simulink model "E5_1_Harmonicas"  (R2018a)
settings: Solver=VariableStepAuto  StartTime=0.0  StopTime=1  RelTol=1e-3
libraries: powerlib x109
settings Model: Creator=Rafael Pavan  LastModifiedBy=Rafael Pavan

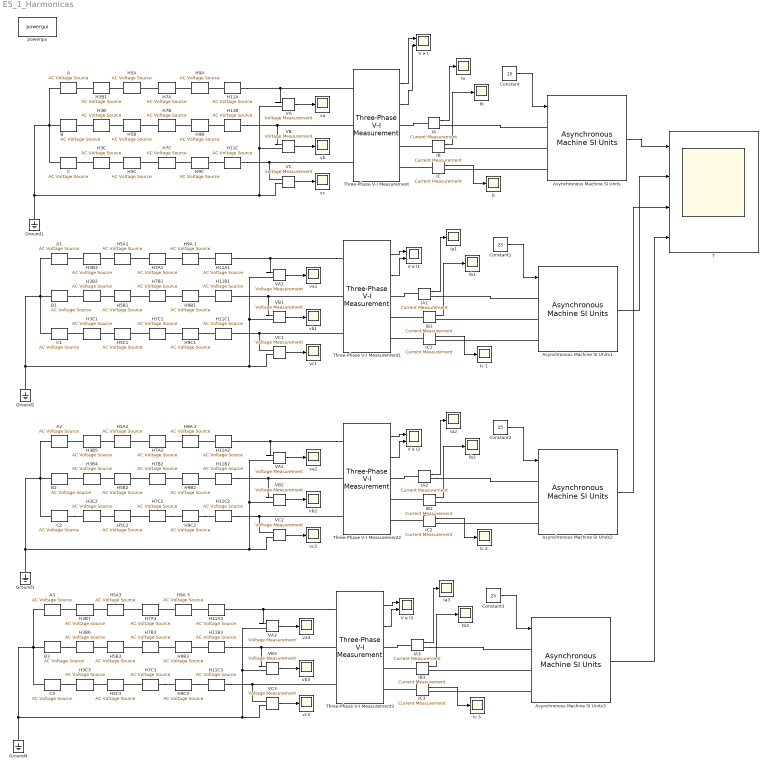
== system E5_1_Harmonicas ==
  A{,1..3} (4 alike) : powerlib/Electrical Sources/AC Voltage Source  Amplitude=179.605  Phase=0  Frequency=60  SampleTime=0  Measurements=None  BusType=PV  Pref=100e4  Qref=0  Qmin=-inf  Qmax=+inf
  Asynchronous Machine SI Units{,1..3} (4 alike) : powerlib/Machines/Asynchronous Machine SI Units  RotorType=Squirrel-cage  PresetModel=No  MechanicalLoad=Torque Tm  ShowDetailedParameters=on  ReferenceFrame=Rotor  Units=SI  MeasurementBus=off  NominalParameters=[38105 220 60]  Stator=[0.5968 0.0003495]  Rotor=[0.6258 0.005473]  Cage1=[0.4155 0.002066]  Cage2=[0.4168 0.0003495]  Lm=0.0354  Mechanical=[0.05 0.005879 3]  PolePairs=2  InitialConditions=[0.03 0 0 0 0 0 0 0]  SimulateSaturation=off  Saturation=[14.03593122, 27.81365428, 53.79336849, 72.68890987, 97.98006896, 148.6815601, 215.7428561, 302.9841135, 428.7778367 ; 230, 322, 414, 460, 506, 552, 598, 644, 690]  LoadFlowParameters=1492000  TsPowergui=0  TsBlock=-1  IterativeModel=Trapezoidal non iterative  IterativeDiscreteModel=Trapezoidal non iterative  Pmec=29150
  B{,1..3} (4 alike) : powerlib/Electrical Sources/AC Voltage Source  Amplitude=179.605  Phase=-120  Frequency=60  SampleTime=0  Measurements=None  BusType=PV  Pref=100e4  Qref=0  Qmin=-inf  Qmax=+inf
  C{,1..3} (4 alike) : powerlib/Electrical Sources/AC Voltage Source  Amplitude=179.605  Phase=120  Frequency=60  SampleTime=0  Measurements=None  BusType=PV  Pref=100e4  Qref=0  Qmin=-inf  Qmax=+inf
  Constant{,1..3} (4 alike) : Constant  Value=25
  Ground{1..4} (4 alike) : powerlib/Elements/Ground  LConnTagsString=a
  H11A : powerlib/Electrical Sources/AC Voltage Source  Amplitude=0  Phase=0  Frequency=660  SampleTime=0  Measurements=None  BusType=PV  Pref=100e4  Qref=0  Qmin=-inf  Qmax=+inf
  H11A1 : powerlib/Electrical Sources/AC Voltage Source  Amplitude=0  Phase=0  Frequency=660  SampleTime=0  Measurements=None  BusType=PV  Pref=100e4  Qref=0  Qmin=-inf  Qmax=+inf
  H11A2 : powerlib/Electrical Sources/AC Voltage Source  Amplitude=179.605*10/100  Phase=0  Frequency=660  SampleTime=0  Measurements=None  BusType=PV  Pref=100e4  Qref=0  Qmin=-inf  Qmax=+inf
  H11A3 : powerlib/Electrical Sources/AC Voltage Source  Amplitude=179.605*5/100  Phase=0  Frequency=660  SampleTime=0  Measurements=None  BusType=PV  Pref=100e4  Qref=0  Qmin=-inf  Qmax=+inf
  H11B : powerlib/Electrical Sources/AC Voltage Source  Amplitude=0  Phase=-120*11  Frequency=660  SampleTime=0  Measurements=None  BusType=PV  Pref=100e4  Qref=0  Qmin=-inf  Qmax=+inf
  H11B1 : powerlib/Electrical Sources/AC Voltage Source  Amplitude=0  Phase=-120*11  Frequency=660  SampleTime=0  Measurements=None  BusType=PV  Pref=100e4  Qref=0  Qmin=-inf  Qmax=+inf
  H11B2 : powerlib/Electrical Sources/AC Voltage Source  Amplitude=179.605*10/100  Phase=-120*11  Frequency=660  SampleTime=0  Measurements=None  BusType=PV  Pref=100e4  Qref=0  Qmin=-inf  Qmax=+inf
  H11B3 : powerlib/Electrical Sources/AC Voltage Source  Amplitude=179.605*5/100  Phase=-120*11  Frequency=660  SampleTime=0  Measurements=None  BusType=PV  Pref=100e4  Qref=0  Qmin=-inf  Qmax=+inf
  H11C : powerlib/Electrical Sources/AC Voltage Source  Amplitude=0  Phase=120*11  Frequency=660  SampleTime=0  Measurements=None  BusType=PV  Pref=100e4  Qref=0  Qmin=-inf  Qmax=+inf
  H11C1 : powerlib/Electrical Sources/AC Voltage Source  Amplitude=0  Phase=120*11  Frequency=660  SampleTime=0  Measurements=None  BusType=PV  Pref=100e4  Qref=0  Qmin=-inf  Qmax=+inf
  H11C2 : powerlib/Electrical Sources/AC Voltage Source  Amplitude=179.605*10/100  Phase=120*11  Frequency=660  SampleTime=0  Measurements=None  BusType=PV  Pref=100e4  Qref=0  Qmin=-inf  Qmax=+inf
  H11C3 : powerlib/Electrical Sources/AC Voltage Source  Amplitude=179.605*5/100  Phase=120*11  Frequency=660  SampleTime=0  Measurements=None  BusType=PV  Pref=100e4  Qref=0  Qmin=-inf  Qmax=+inf
  H3B : powerlib/Electrical Sources/AC Voltage Source  Amplitude=179.605*10/100  Phase=-120*3  Frequency=180  SampleTime=0  Measurements=None  BusType=PV  Pref=100e4  Qref=0  Qmin=-inf  Qmax=+inf
  H3B1 : powerlib/Electrical Sources/AC Voltage Source  Amplitude=179.605*10/100  Phase=0*3  Frequency=60*3  SampleTime=0  Measurements=None  BusType=PV  Pref=100e4  Qref=0  Qmin=-inf  Qmax=+inf
  H3B2 : powerlib/Electrical Sources/AC Voltage Source  Amplitude=0  Phase=-120*3  Frequency=180  SampleTime=0  Measurements=None  BusType=PV  Pref=100e4  Qref=0  Qmin=-inf  Qmax=+inf
  H3B3 : powerlib/Electrical Sources/AC Voltage Source  Amplitude=0  Phase=0*3  Frequency=60*3  SampleTime=0  Measurements=None  BusType=PV  Pref=100e4  Qref=0  Qmin=-inf  Qmax=+inf
  H3B4 : powerlib/Electrical Sources/AC Voltage Source  Amplitude=0  Phase=-120*3  Frequency=180  SampleTime=0  Measurements=None  BusType=PV  Pref=100e4  Qref=0  Qmin=-inf  Qmax=+inf
  H3B5 : powerlib/Electrical Sources/AC Voltage Source  Amplitude=0  Phase=0*3  Frequency=60*3  SampleTime=0  Measurements=None  BusType=PV  Pref=100e4  Qref=0  Qmin=-inf  Qmax=+inf
  H3B6 : powerlib/Electrical Sources/AC Voltage Source  Amplitude=0  Phase=-120*3  Frequency=180  SampleTime=0  Measurements=None  BusType=PV  Pref=100e4  Qref=0  Qmin=-inf  Qmax=+inf
  H3B7 : powerlib/Electrical Sources/AC Voltage Source  Amplitude=0  Phase=0*3  Frequency=60*3  SampleTime=0  Measurements=None  BusType=PV  Pref=100e4  Qref=0  Qmin=-inf  Qmax=+inf
  H3C : powerlib/Electrical Sources/AC Voltage Source  Amplitude=179.605*10/100  Phase=120*3  Frequency=180  SampleTime=0  Measurements=None  BusType=PV  Pref=100e4  Qref=0  Qmin=-inf  Qmax=+inf
  H3C1 : powerlib/Electrical Sources/AC Voltage Source  Amplitude=0  Phase=120*3  Frequency=180  SampleTime=0  Measurements=None  BusType=PV  Pref=100e4  Qref=0  Qmin=-inf  Qmax=+inf
  H3C2 : powerlib/Electrical Sources/AC Voltage Source  Amplitude=0  Phase=120*3  Frequency=180  SampleTime=0  Measurements=None  BusType=PV  Pref=100e4  Qref=0  Qmin=-inf  Qmax=+inf
  H3C3 : powerlib/Electrical Sources/AC Voltage Source  Amplitude=0  Phase=120*3  Frequency=180  SampleTime=0  Measurements=None  BusType=PV  Pref=100e4  Qref=0  Qmin=-inf  Qmax=+inf
  H5A : powerlib/Electrical Sources/AC Voltage Source  Amplitude=0  Phase=0  Frequency=300  SampleTime=0  Measurements=None  BusType=PV  Pref=100e4  Qref=0  Qmin=-inf  Qmax=+inf
  H5A1 : powerlib/Electrical Sources/AC Voltage Source  Amplitude=0  Phase=0  Frequency=300  SampleTime=0  Measurements=None  BusType=PV  Pref=100e4  Qref=0  Qmin=-inf  Qmax=+inf
  H5A2 : powerlib/Electrical Sources/AC Voltage Source  Amplitude=179.605*10/100  Phase=0  Frequency=300  SampleTime=0  Measurements=None  BusType=PV  Pref=100e4  Qref=0  Qmin=-inf  Qmax=+inf
  H5A3 : powerlib/Electrical Sources/AC Voltage Source  Amplitude=179.605*5/100  Phase=0  Frequency=300  SampleTime=0  Measurements=None  BusType=PV  Pref=100e4  Qref=0  Qmin=-inf  Qmax=+inf
  H5B : powerlib/Electrical Sources/AC Voltage Source  Amplitude=0  Phase=-120*5  Frequency=300  SampleTime=0  Measurements=None  BusType=PV  Pref=100e4  Qref=0  Qmin=-inf  Qmax=+inf
  H5B1 : powerlib/Electrical Sources/AC Voltage Source  Amplitude=0  Phase=-120*5  Frequency=300  SampleTime=0  Measurements=None  BusType=PV  Pref=100e4  Qref=0  Qmin=-inf  Qmax=+inf
  H5B2 : powerlib/Electrical Sources/AC Voltage Source  Amplitude=179.605*10/100  Phase=-120*5  Frequency=300  SampleTime=0  Measurements=None  BusType=PV  Pref=100e4  Qref=0  Qmin=-inf  Qmax=+inf
  H5B3 : powerlib/Electrical Sources/AC Voltage Source  Amplitude=179.605*5/100  Phase=-120*5  Frequency=300  SampleTime=0  Measurements=None  BusType=PV  Pref=100e4  Qref=0  Qmin=-inf  Qmax=+inf
  H5C : powerlib/Electrical Sources/AC Voltage Source  Amplitude=0  Phase=120*5  Frequency=300  SampleTime=0  Measurements=None  BusType=PV  Pref=100e4  Qref=0  Qmin=-inf  Qmax=+inf
  H5C1 : powerlib/Electrical Sources/AC Voltage Source  Amplitude=0  Phase=120*5  Frequency=300  SampleTime=0  Measurements=None  BusType=PV  Pref=100e4  Qref=0  Qmin=-inf  Qmax=+inf
  H5C2 : powerlib/Electrical Sources/AC Voltage Source  Amplitude=179.605*10/100  Phase=120*5  Frequency=300  SampleTime=0  Measurements=None  BusType=PV  Pref=100e4  Qref=0  Qmin=-inf  Qmax=+inf
  H5C3 : powerlib/Electrical Sources/AC Voltage Source  Amplitude=179.605*5/100  Phase=120*5  Frequency=300  SampleTime=0  Measurements=None  BusType=PV  Pref=100e4  Qref=0  Qmin=-inf  Qmax=+inf
  H7A : powerlib/Electrical Sources/AC Voltage Source  Amplitude=0  Phase=0  Frequency=420  SampleTime=0  Measurements=None  BusType=PV  Pref=100e4  Qref=0  Qmin=-inf  Qmax=+inf
  H7A1 : powerlib/Electrical Sources/AC Voltage Source  Amplitude=179.605*15/100  Phase=0  Frequency=420  SampleTime=0  Measurements=None  BusType=PV  Pref=100e4  Qref=0  Qmin=-inf  Qmax=+inf
  H7A2 : powerlib/Electrical Sources/AC Voltage Source  Amplitude=0  Phase=0  Frequency=420  SampleTime=0  Measurements=None  BusType=PV  Pref=100e4  Qref=0  Qmin=-inf  Qmax=+inf
  H7A3 : powerlib/Electrical Sources/AC Voltage Source  Amplitude=179.605*7/100  Phase=0  Frequency=420  SampleTime=0  Measurements=None  BusType=PV  Pref=100e4  Qref=0  Qmin=-inf  Qmax=+inf
  H7B : powerlib/Electrical Sources/AC Voltage Source  Amplitude=0  Phase=-120*7  Frequency=420  SampleTime=0  Measurements=None  BusType=PV  Pref=100e4  Qref=0  Qmin=-inf  Qmax=+inf
  H7B1 : powerlib/Electrical Sources/AC Voltage Source  Amplitude=179.605*15/100  Phase=-120*7  Frequency=420  SampleTime=0  Measurements=None  BusType=PV  Pref=100e4  Qref=0  Qmin=-inf  Qmax=+inf
  H7B2 : powerlib/Electrical Sources/AC Voltage Source  Amplitude=0  Phase=-120*7  Frequency=420  SampleTime=0  Measurements=None  BusType=PV  Pref=100e4  Qref=0  Qmin=-inf  Qmax=+inf
  H7B3 : powerlib/Electrical Sources/AC Voltage Source  Amplitude=179.605*7/100  Phase=-120*7  Frequency=420  SampleTime=0  Measurements=None  BusType=PV  Pref=100e4  Qref=0  Qmin=-inf  Qmax=+inf
  H7C : powerlib/Electrical Sources/AC Voltage Source  Amplitude=0  Phase=120*7  Frequency=420  SampleTime=0  Measurements=None  BusType=PV  Pref=100e4  Qref=0  Qmin=-inf  Qmax=+inf
  H7C1 : powerlib/Electrical Sources/AC Voltage Source  Amplitude=179.605*15/100  Phase=120*7  Frequency=420  SampleTime=0  Measurements=None  BusType=PV  Pref=100e4  Qref=0  Qmin=-inf  Qmax=+inf
  H7C2 : powerlib/Electrical Sources/AC Voltage Source  Amplitude=0  Phase=120*7  Frequency=420  SampleTime=0  Measurements=None  BusType=PV  Pref=100e4  Qref=0  Qmin=-inf  Qmax=+inf
  H7C3 : powerlib/Electrical Sources/AC Voltage Source  Amplitude=179.605*7/100  Phase=120*7  Frequency=420  SampleTime=0  Measurements=None  BusType=PV  Pref=100e4  Qref=0  Qmin=-inf  Qmax=+inf
  "H9A " : powerlib/Electrical Sources/AC Voltage Source  Amplitude=179.605*5/100  Phase=0  Frequency=540  SampleTime=0  Measurements=None  BusType=PV  Pref=100e4  Qref=0  Qmin=-inf  Qmax=+inf
  H9A 1 : powerlib/Electrical Sources/AC Voltage Source  Amplitude=0  Phase=0  Frequency=540  SampleTime=0  Measurements=None  BusType=PV  Pref=100e4  Qref=0  Qmin=-inf  Qmax=+inf
  H9A 2 : powerlib/Electrical Sources/AC Voltage Source  Amplitude=0  Phase=0  Frequency=540  SampleTime=0  Measurements=None  BusType=PV  Pref=100e4  Qref=0  Qmin=-inf  Qmax=+inf
  H9A 3 : powerlib/Electrical Sources/AC Voltage Source  Amplitude=0  Phase=0  Frequency=540  SampleTime=0  Measurements=None  BusType=PV  Pref=100e4  Qref=0  Qmin=-inf  Qmax=+inf
  H9B : powerlib/Electrical Sources/AC Voltage Source  Amplitude=179.605*5/100  Phase=-120*9  Frequency=540  SampleTime=0  Measurements=None  BusType=PV  Pref=100e4  Qref=0  Qmin=-inf  Qmax=+inf
  H9B1 : powerlib/Electrical Sources/AC Voltage Source  Amplitude=0  Phase=-120*9  Frequency=540  SampleTime=0  Measurements=None  BusType=PV  Pref=100e4  Qref=0  Qmin=-inf  Qmax=+inf
  H9B2 : powerlib/Electrical Sources/AC Voltage Source  Amplitude=0  Phase=-120*9  Frequency=540  SampleTime=0  Measurements=None  BusType=PV  Pref=100e4  Qref=0  Qmin=-inf  Qmax=+inf
  H9B3 : powerlib/Electrical Sources/AC Voltage Source  Amplitude=0  Phase=-120*9  Frequency=540  SampleTime=0  Measurements=None  BusType=PV  Pref=100e4  Qref=0  Qmin=-inf  Qmax=+inf
  H9C : powerlib/Electrical Sources/AC Voltage Source  Amplitude=179.605*5/100  Phase=120*9  Frequency=540  SampleTime=0  Measurements=None  BusType=PV  Pref=100e4  Qref=0  Qmin=-inf  Qmax=+inf
  H9C1 : powerlib/Electrical Sources/AC Voltage Source  Amplitude=0  Phase=120*9  Frequency=540  SampleTime=0  Measurements=None  BusType=PV  Pref=100e4  Qref=0  Qmin=-inf  Qmax=+inf
  H9C2 : powerlib/Electrical Sources/AC Voltage Source  Amplitude=0  Phase=120*9  Frequency=540  SampleTime=0  Measurements=None  BusType=PV  Pref=100e4  Qref=0  Qmin=-inf  Qmax=+inf
  H9C3 : powerlib/Electrical Sources/AC Voltage Source  Amplitude=0  Phase=120*9  Frequency=540  SampleTime=0  Measurements=None  BusType=PV  Pref=100e4  Qref=0  Qmin=-inf  Qmax=+inf
  IA{,1..3} (4 alike) : powerlib/Measurements/Current Measurement  PhasorSimulation=off  OutputType=Complex  PSBequivalent=0
  IB{,1..3} (4 alike) : powerlib/Measurements/Current Measurement  PhasorSimulation=off  OutputType=Complex  PSBequivalent=0
  IC{,1..3} (4 alike) : powerlib/Measurements/Current Measurement  PhasorSimulation=off  OutputType=Complex  PSBequivalent=0
  Ia{,1..3} (4 alike) : Scope
  Ib{,1..3} (4 alike) : Scope
  Ic {,1..3} (4 alike) : Scope
  T : Scope  NumInputPorts=4
  Three-Phase V-I Measurement{,1..3} (4 alike) : powerlib/Measurements/Three-Phase V-I Measurement  VoltageMeasurement=phase-to-ground  SetLabelV=off  LabelV=Vabc  Vpu=off  VpuLL=off  CurrentMeasurement=yes  SetLabelI=off  LabelI=Iabc  Ipu=off  Pbase=100e6  Vbase=500e3  OutputType=Complex  PhasorSimulation=off  PSBequivalent=0
  V e I{,1..3} (4 alike) : Scope  NumInputPorts=2
  VA{,1..3} (4 alike) : powerlib/Measurements/Voltage Measurement  PhasorSimulation=off  OutputType=Complex  PSBequivalent=0
  VB{,1..3} (4 alike) : powerlib/Measurements/Voltage Measurement  PhasorSimulation=off  OutputType=Complex  PSBequivalent=0
  VC{,1..3} (4 alike) : powerlib/Measurements/Voltage Measurement  PhasorSimulation=off  OutputType=Complex  PSBequivalent=0
  powergui : powerlib/powergui  Priority=1  SimulationMode=Continuous  SampleTime=50e-6  frequency=60  Iterations=50  frequencyindice=60  Pbase=100e6  ErrMax=1e-4  UnitsV=kV  UnitsW=MW  buscounter=0  FunctionMessages=on  echomessages=off  EnableUseOfTLC=off  CurrentSourceSwitches=off  DisableSnubberDevices=off  DisableRonSwitches=off  DisableVfSwitches=off  DisplayEquations=off  SolverType=Tustin/Backward Euler (TBE)  Interpol=off  ExternalGateDelay=off  methode=off  Ts=100  x0status=blocks  SPID=on  SwTol=0  HookPort=off  RestoreLinks=warning  ResistiveCurrentMeasurement=off  Frange=[0:2:500]  Ylog=off  Xlog=on  ShowGrid=off  save=off  variable=ZData  structure=ia3  ZoomFFT=off  StartTime=0.2  cycles=12  DisplayStyle=1  fundamental=60  FreqAxis=off  MaxFrequency=1000  frequencyindicesteady=1  RmsSteady=2  display=off
  va{,1..3} (4 alike) : Scope
  vb{,1..3} (4 alike) : Scope
  vc{,1..3} (4 alike) : Scope
  wires:
  VA/1 -> va/1
  VB/1 -> vb/1
  VC/1 -> vc/1
  Three-Phase V-I Measurement/1 -> V e I/1
  IA/1 -> Ia/1
  IB/1 -> Ib/1
  IC/1 -> "Ic "/1
  Asynchronous Machine SI Units/1 -> T/1
  Constant/1 -> Asynchronous Machine SI Units/1
  Three-Phase V-I Measurement/2 -> V e I/2
  Three-Phase V-I Measurement1/2 -> V e I1/2
  Constant1/1 -> Asynchronous Machine SI Units1/1
  IB1/1 -> Ib1/1
  VC1/1 -> vc1/1
  Three-Phase V-I Measurement1/1 -> V e I1/1
  IA1/1 -> Ia1/1
  IC1/1 -> Ic 1/1
  VA1/1 -> va1/1
  VB1/1 -> vb1/1
  Asynchronous Machine SI Units1/1 -> T/2
  Three-Phase V-I Measurement2/1 -> V e I2/1
  VA2/1 -> va2/1
  Asynchronous Machine SI Units2/1 -> T/3
  IA2/1 -> Ia2/1
  IB2/1 -> Ib2/1
  Constant2/1 -> Asynchronous Machine SI Units2/1
  Three-Phase V-I Measurement2/2 -> V e I2/2
  VB2/1 -> vb2/1
  VC2/1 -> vc2/1
  IC2/1 -> Ic 2/1
  Three-Phase V-I Measurement3/1 -> V e I3/1
  VA3/1 -> va3/1
  Asynchronous Machine SI Units3/1 -> T/4
  IA3/1 -> Ia3/1
  IB3/1 -> Ib3/1
  Constant3/1 -> Asynchronous Machine SI Units3/1
  Three-Phase V-I Measurement3/2 -> V e I3/2
  VB3/1 -> vb3/1
  VC3/1 -> vc3/1
  IC3/1 -> Ic 3/1
  connections:
  A/LConn1 -- C/LConn1 -- B/LConn1 -- VA/LConn2 -- VB/LConn2 -- VC/LConn2 -- Ground1/LConn1
  H3B1/LConn1 -- A/RConn1
  B/RConn1 -- H3B/LConn1
  C/RConn1 -- H3C/LConn1
  H11C/RConn1 -- VC/LConn1 -- Three-Phase V-I Measurement/LConn3
  H11B/RConn1 -- VB/LConn1 -- Three-Phase V-I Measurement/LConn2
  H5A/LConn1 -- H3B1/RConn1
  H7B/LConn1 -- H5B/RConn1
  H5C/LConn1 -- H3C/RConn1
  H7A/LConn1 -- H5A/RConn1
  "H9A "/LConn1 -- H7A/RConn1
  H5B/LConn1 -- H3B/RConn1
  H11B/LConn1 -- H9B/RConn1
  H7C/LConn1 -- H5C/RConn1
  H9B/LConn1 -- H7B/RConn1
  H9C/RConn1 -- H11C/LConn1
  H11A/LConn1 -- "H9A "/RConn1
  H7C/RConn1 -- H9C/LConn1
  H11A/RConn1 -- VA/LConn1 -- Three-Phase V-I Measurement/LConn1
  IA/LConn1 -- Three-Phase V-I Measurement/RConn1
  IB/LConn1 -- Three-Phase V-I Measurement/RConn2
  IC/LConn1 -- Three-Phase V-I Measurement/RConn3
  Asynchronous Machine SI Units/LConn2 -- IB/RConn1
  IA/RConn1 -- Asynchronous Machine SI Units/LConn1
  Asynchronous Machine SI Units/LConn3 -- IC/RConn1
  VB1/LConn2 -- Ground2/LConn1 -- C1/LConn1 -- B1/LConn1 -- A1/LConn1 -- VC1/LConn2 -- VA1/LConn2
  H11B1/RConn1 -- VB1/LConn1 -- Three-Phase V-I Measurement1/LConn2
  Three-Phase V-I Measurement1/LConn1 -- H11A1/RConn1 -- VA1/LConn1
  H11C1/RConn1 -- VC1/LConn1 -- Three-Phase V-I Measurement1/LConn3
  Asynchronous Machine SI Units1/LConn2 -- IB1/RConn1
  IA1/LConn1 -- Three-Phase V-I Measurement1/RConn1
  Asynchronous Machine SI Units1/LConn3 -- IC1/RConn1
  H7B1/LConn1 -- H5B1/RConn1
  IA1/RConn1 -- Asynchronous Machine SI Units1/LConn1
  H7C1/RConn1 -- H9C1/LConn1
  IB1/LConn1 -- Three-Phase V-I Measurement1/RConn2
  H5B1/LConn1 -- H3B2/RConn1
  H3B3/LConn1 -- A1/RConn1
  H11B1/LConn1 -- H9B1/RConn1
  IC1/LConn1 -- Three-Phase V-I Measurement1/RConn3
  H9A 1/LConn1 -- H7A1/RConn1
  H9C1/RConn1 -- H11C1/LConn1
  H7C1/LConn1 -- H5C1/RConn1
  H5A1/LConn1 -- H3B3/RConn1
  H11A1/LConn1 -- H9A 1/RConn1
  H5C1/LConn1 -- H3C1/RConn1
  B1/RConn1 -- H3B2/LConn1
  H9B1/LConn1 -- H7B1/RConn1
  H7A1/LConn1 -- H5A1/RConn1
  C1/RConn1 -- H3C1/LConn1
  H11C2/RConn1 -- VC2/LConn1 -- Three-Phase V-I Measurement2/LConn3
  VB2/LConn2 -- VA2/LConn2 -- Ground3/LConn1 -- C2/LConn1 -- B2/LConn1 -- A2/LConn1 -- VC2/LConn2
  Three-Phase V-I Measurement2/LConn1 -- H11A2/RConn1 -- VA2/LConn1
  H11B2/RConn1 -- VB2/LConn1 -- Three-Phase V-I Measurement2/LConn2
  H5C2/LConn1 -- H3C2/RConn1
  H5A2/LConn1 -- H3B5/RConn1
  IA2/RConn1 -- Asynchronous Machine SI Units2/LConn1
  H9B2/LConn1 -- H7B2/RConn1
  H9A 2/LConn1 -- H7A2/RConn1
  B2/RConn1 -- H3B4/LConn1
  H3B5/LConn1 -- A2/RConn1
  C2/RConn1 -- H3C2/LConn1
  IB2/LConn1 -- Three-Phase V-I Measurement2/RConn2
  H5B2/LConn1 -- H3B4/RConn1
  H7A2/LConn1 -- H5A2/RConn1
  Asynchronous Machine SI Units2/LConn2 -- IB2/RConn1
  H7C2/RConn1 -- H9C2/LConn1
  Asynchronous Machine SI Units2/LConn3 -- IC2/RConn1
  IA2/LConn1 -- Three-Phase V-I Measurement2/RConn1
  H9C2/RConn1 -- H11C2/LConn1
  H7C2/LConn1 -- H5C2/RConn1
  H11A2/LConn1 -- H9A 2/RConn1
  IC2/LConn1 -- Three-Phase V-I Measurement2/RConn3
  H11B2/LConn1 -- H9B2/RConn1
  H7B2/LConn1 -- H5B2/RConn1
  H11C3/RConn1 -- VC3/LConn1 -- Three-Phase V-I Measurement3/LConn3
  VB3/LConn2 -- VA3/LConn2 -- Ground4/LConn1 -- C3/LConn1 -- B3/LConn1 -- A3/LConn1 -- VC3/LConn2
  Three-Phase V-I Measurement3/LConn1 -- H11A3/RConn1 -- VA3/LConn1
  H11B3/RConn1 -- VB3/LConn1 -- Three-Phase V-I Measurement3/LConn2
  H5C3/LConn1 -- H3C3/RConn1
  H5A3/LConn1 -- H3B7/RConn1
  IA3/RConn1 -- Asynchronous Machine SI Units3/LConn1
  H9B3/LConn1 -- H7B3/RConn1
  H9A 3/LConn1 -- H7A3/RConn1
  B3/RConn1 -- H3B6/LConn1
  H3B7/LConn1 -- A3/RConn1
  C3/RConn1 -- H3C3/LConn1
  IB3/LConn1 -- Three-Phase V-I Measurement3/RConn2
  H5B3/LConn1 -- H3B6/RConn1
  H7A3/LConn1 -- H5A3/RConn1
  Asynchronous Machine SI Units3/LConn2 -- IB3/RConn1
  H7C3/RConn1 -- H9C3/LConn1
  Asynchronous Machine SI Units3/LConn3 -- IC3/RConn1
  IA3/LConn1 -- Three-Phase V-I Measurement3/RConn1
  H9C3/RConn1 -- H11C3/LConn1
  H7C3/LConn1 -- H5C3/RConn1
  H11A3/LConn1 -- H9A 3/RConn1
  IC3/LConn1 -- Three-Phase V-I Measurement3/RConn3
  H11B3/LConn1 -- H9B3/RConn1
  H7B3/LConn1 -- H5B3/RConn1
